simulink model "dois"  (R2022b)
settings: Solver=VariableStepAuto  StartTime=0.0  StopTime=10.0  RelTol=1e-3
settings Model: Creator=Admin  LastModifiedBy=Admin

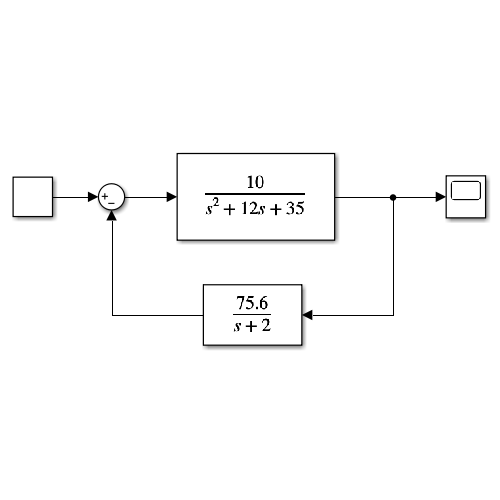
[thumbnail: Simulink's stored preview of the top-level diagram]
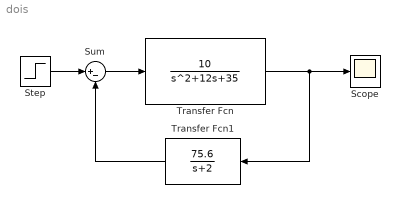
== system dois ==
  Scope : Scope
  Step : Step  SampleTime=0
  Sum : Sum  Inputs=|+-
  Transfer Fcn : TransferFcn  Numerator=[10]  Denominator=[1 12 35]
  Transfer Fcn1 : TransferFcn  Numerator=[75.6]  Denominator=[1 2]
  wires:
  Transfer Fcn/1 -> Transfer Fcn1/1, Scope/1
  Sum/1 -> Transfer Fcn/1
  Transfer Fcn1/1 -> Sum/2
  Step/1 -> Sum/1
